simulink model "narx"  (R2019a)
(part 6 of 6)

  "IW{2,1}(60,:)'" : Constant  Value=[0.5846270390584165088654344799579121172428131103515625;0.325648571693005040028623398029594682157039642333984375;-1.1173501219859260924494037681142799556255340576171875;-0.51463684804933806926641182144521735608577728271484375;-0.57361062364307213723435552310547791421413421630859375;-1.3326939837995581683571799658238887786865234375;0.281281193943799745493805630758288316428661346435546875;-0.85669198049516370740974480213481001555919647216796875;0.047948586779547490432928924519728752784430980682373046875;0.90428829582249170560004358776495791971683502197265625]
      mask Display: e = 0.06;c1 = [120 150 230]/255;c2 = ([120 150 230]+0)/383;c3 = ([120 150 230]+128)/383;patch([0 1 1 0],[0 0 1 1],c1);patch([0 1 1 1-e 1-e 0+e],[0 0 1 1-e 0+e 0+e],c2);patch([0 0 1 1-e 0+e 0+e],[0 1 1 1-e 1-e 0+e],c3);plot([0 1 1 0 0],[0 0 1 1 0]);disp('weights');
  "IW{2,1}(61,:)'" : Constant  Value=[0.78103658740860038012243649063748307526111602783203125;1.3860771911427054448040507850237190723419189453125;-0.451371320114015983637756335156154818832874298095703125;-0.335541633513115444831242939471849240362644195556640625;-1.51059236681972119953343280940316617488861083984375;-0.057469963340264003381907542689077672548592090606689453125;1.3584626519773010944192037641187198460102081298828125;-0.629676215555289520153792182100005447864532470703125;-0.60136172032273271792490731968428008258342742919921875;0.9730549079016139746300950719160027801990509033203125]
      mask Display: e = 0.06;c1 = [120 150 230]/255;c2 = ([120 150 230]+0)/383;c3 = ([120 150 230]+128)/383;patch([0 1 1 0],[0 0 1 1],c1);patch([0 1 1 1-e 1-e 0+e],[0 0 1 1-e 0+e 0+e],c2);patch([0 0 1 1-e 0+e 0+e],[0 1 1 1-e 1-e 0+e],c3);plot([0 1 1 0 0],[0 0 1 1 0]);disp('weights');
  "IW{2,1}(62,:)'" : Constant  Value=[0.04940523944418449830973116831955849193036556243896484375;0.63038937153419549730415383237414062023162841796875;-0.400671943461981261425108868934330530464649200439453125;-0.3260626963057704497117583741783164441585540771484375;-1.4699748324566976886984548400505445897579193115234375;-0.52485565032367464954887736894306726753711700439453125;0.52077193033993662840686056370032019913196563720703125;-1.41959117855626715254402370192110538482666015625;-0.61414649132420906507690006037591956555843353271484375;0.9727704163309398577297315569012425839900970458984375]
      mask Display: e = 0.06;c1 = [120 150 230]/255;c2 = ([120 150 230]+0)/383;c3 = ([120 150 230]+128)/383;patch([0 1 1 0],[0 0 1 1],c1);patch([0 1 1 1-e 1-e 0+e],[0 0 1 1-e 0+e 0+e],c2);patch([0 0 1 1-e 0+e 0+e],[0 1 1 1-e 1-e 0+e],c3);plot([0 1 1 0 0],[0 0 1 1 0]);disp('weights');
  "IW{2,1}(63,:)'" : Constant  Value=[0.231719668878419382540556625826866365969181060791015625;0.15579981414367771730411504904623143374919891357421875;-1.133213915627591550361330519081093370914459228515625;-1.01533686843544668221284155151806771755218505859375;-0.5337548818325708044341126878862269222736358642578125;-1.0275630873972179113451375087606720626354217529296875;0.31528407357524856902131205060868524014949798583984375;-0.90450554307037889234521799153299070894718170166015625;-0.80580912230389356576409909393987618386745452880859375;0.902204107924529097317645209841430187225341796875]
      mask Display: e = 0.06;c1 = [120 150 230]/255;c2 = ([120 150 230]+0)/383;c3 = ([120 150 230]+128)/383;patch([0 1 1 0],[0 0 1 1],c1);patch([0 1 1 1-e 1-e 0+e],[0 0 1 1-e 0+e 0+e],c2);patch([0 0 1 1-e 0+e 0+e],[0 1 1 1-e 1-e 0+e],c3);plot([0 1 1 0 0],[0 0 1 1 0]);disp('weights');
  "IW{2,1}(64,:)'" : Constant  Value=[1.0877443347215358659951789377373643219470977783203125;1.193166973587330037531728521571494638919830322265625;-0.42455721543596547373766725286259315907955169677734375;-1.4617036935264919872423661217908374965190887451171875;-1.2080926119362305204418817083933390676975250244140625;-1.0557409686524616976299739690148271620273590087890625;0.365292773089297584387935557970195077359676361083984375;-0.9730446570433100017538663450977765023708343505859375;-0.61090531142060966462992155356914736330509185791015625;0.7703918279306207761436553482781164348125457763671875]
      mask Display: e = 0.06;c1 = [120 150 230]/255;c2 = ([120 150 230]+0)/383;c3 = ([120 150 230]+128)/383;patch([0 1 1 0],[0 0 1 1],c1);patch([0 1 1 1-e 1-e 0+e],[0 0 1 1-e 0+e 0+e],c2);patch([0 0 1 1-e 0+e 0+e],[0 1 1 1-e 1-e 0+e],c3);plot([0 1 1 0 0],[0 0 1 1 0]);disp('weights');
  "IW{2,1}(65,:)'" : Constant  Value=[0.68003601989002981920151569283916614949703216552734375;0.6639319036035191690103829387226141989231109619140625;-0.442406882331512762984715436687110923230648040771484375;-0.55502664647763122474088959279470145702362060546875;-1.43356712752413528733086423017084598541259765625;-0.269969187207295846508969816568423993885517120361328125;1.0574225063279472092148125739186070859432220458984375;-0.78837674667073809331441225367598235607147216796875;-0.5927181169921771353159556383616290986537933349609375;0.93202374184012481972416708231321536004543304443359375]
      mask Display: e = 0.06;c1 = [120 150 230]/255;c2 = ([120 150 230]+0)/383;c3 = ([120 150 230]+128)/383;patch([0 1 1 0],[0 0 1 1],c1);patch([0 1 1 1-e 1-e 0+e],[0 0 1 1-e 0+e 0+e],c2);patch([0 0 1 1-e 0+e 0+e],[0 1 1 1-e 1-e 0+e],c3);plot([0 1 1 0 0],[0 0 1 1 0]);disp('weights');
  "IW{2,1}(66,:)'" : Constant  Value=[0.9744306052910489679419470121501944959163665771484375;0.194329386895280009639463969506323337554931640625;-0.893551305415250407548910516197793185710906982421875;-1.70839989126382629791578438016586005687713623046875;-0.563425857602368740373321998049505054950714111328125;-0.76580929707367972891773888477473519742488861083984375;0.7410351670580634930729502229951322078704833984375;-0.9051439688157305596405421965755522251129150390625;0.024835755139511590805501128897958551533520221710205078125;0.720062910865631788936980228754691779613494873046875]
      mask Display: e = 0.06;c1 = [120 150 230]/255;c2 = ([120 150 230]+0)/383;c3 = ([120 150 230]+128)/383;patch([0 1 1 0],[0 0 1 1],c1);patch([0 1 1 1-e 1-e 0+e],[0 0 1 1-e 0+e 0+e],c2);patch([0 0 1 1-e 0+e 0+e],[0 1 1 1-e 1-e 0+e],c3);plot([0 1 1 0 0],[0 0 1 1 0]);disp('weights');
  "IW{2,1}(67,:)'" : Constant  Value=[0.795900962746471041242557475925423204898834228515625;-1.031300600699818215133518606307916343212127685546875;-0.95195758629597626576668289999361149966716766357421875;-1.2650340176427172789175301659270189702510833740234375;-0.557486607894674079943797551095485687255859375;-0.74762514462963969297248922885046340525150299072265625;0.71583736946448606186521601557615213096141815185546875;-0.89179256466640433043124858158989809453487396240234375;0.221469013754930721393776593686197884380817413330078125;0.77004158983198767174371823784895241260528564453125]
      mask Display: e = 0.06;c1 = [120 150 230]/255;c2 = ([120 150 230]+0)/383;c3 = ([120 150 230]+128)/383;patch([0 1 1 0],[0 0 1 1],c1);patch([0 1 1 1-e 1-e 0+e],[0 0 1 1-e 0+e 0+e],c2);patch([0 0 1 1-e 0+e 0+e],[0 1 1 1-e 1-e 0+e],c3);plot([0 1 1 0 0],[0 0 1 1 0]);disp('weights');
  "IW{2,1}(68,:)'" : Constant  Value=[0.0784208847591110203012476631556637585163116455078125;1.23349585767250236045811107032932341098785400390625;-0.965344275793105222049916847026906907558441162109375;-0.3986454969972170747638529064715839922428131103515625;-0.80448343689417978197297998121939599514007568359375;-0.048251660507535092115016794878101791255176067352294921875;1.217323065165488937822146908729337155818939208984375;-1.253030776061826667699961035395972430706024169921875;0.0162111061744857620769977302188635803759098052978515625;0.96262616564392489149071252541034482419490814208984375]
      mask Display: e = 0.06;c1 = [120 150 230]/255;c2 = ([120 150 230]+0)/383;c3 = ([120 150 230]+128)/383;patch([0 1 1 0],[0 0 1 1],c1);patch([0 1 1 1-e 1-e 0+e],[0 0 1 1-e 0+e 0+e],c2);patch([0 0 1 1-e 0+e 0+e],[0 1 1 1-e 1-e 0+e],c3);plot([0 1 1 0 0],[0 0 1 1 0]);disp('weights');
  "IW{2,1}(69,:)'" : Constant  Value=[0.051272674564019175835749564384968834929168224334716796875;0.43668213391726939942572016661870293319225311279296875;-1.4605052995373946078672133808140642940998077392578125;-1.3530486090437376933692803504527546465396881103515625;-0.189856659347411582672293661744333803653717041015625;-0.91662647122350671136103983371867798268795013427734375;0.7835348999612705700457127022673375904560089111328125;-0.1301188740913402919208152752617024816572666168212890625;-0.80702164776667240086993615477695129811763763427734375;0.91623960712838059539109281104174442589282989501953125]
      mask Display: e = 0.06;c1 = [120 150 230]/255;c2 = ([120 150 230]+0)/383;c3 = ([120 150 230]+128)/383;patch([0 1 1 0],[0 0 1 1],c1);patch([0 1 1 1-e 1-e 0+e],[0 0 1 1-e 0+e 0+e],c2);patch([0 0 1 1-e 0+e 0+e],[0 1 1 1-e 1-e 0+e],c3);plot([0 1 1 0 0],[0 0 1 1 0]);disp('weights');
  "IW{2,1}(7,:)'" : Constant  Value=[-0.074920241317970426297989661179599352180957794189453125;-0.2477101832749133147881792638145270757377147674560546875;-0.78953000952122776023855976745835505425930023193359375;-0.79576047048455311738734963000752031803131103515625;-1.0322962303491272084698948674486018717288970947265625;0.6771202965445819454970433071139268577098846435546875;1.6734147566400012774323613484739325940608978271484375;-0.91740999359185526618176709234830923378467559814453125;-0.89357860194830951439115551693248562514781951904296875;0.9687525516372412770493838252150453627109527587890625]
      mask Display: e = 0.06;c1 = [120 150 230]/255;c2 = ([120 150 230]+0)/383;c3 = ([120 150 230]+128)/383;patch([0 1 1 0],[0 0 1 1],c1);patch([0 1 1 1-e 1-e 0+e],[0 0 1 1-e 0+e 0+e],c2);patch([0 0 1 1-e 0+e 0+e],[0 1 1 1-e 1-e 0+e],c3);plot([0 1 1 0 0],[0 0 1 1 0]);disp('weights');
  "IW{2,1}(70,:)'" : Constant  Value=[0.40830206338846186664426340939826332032680511474609375;1.3423465582091556047572566967573948204517364501953125;-0.594085903064165865572476832312531769275665283203125;-0.98655841293440060812969250036985613405704498291015625;-1.1832782921037701129307606606744229793548583984375;-1.059393468812497740572098336997441947460174560546875;0.3328600660883704875914190779440104961395263671875;-0.85908977292932420244397917485912330448627471923828125;-0.90237675196684852263473430866724811494350433349609375;0.9041786453484832453142416852642782032489776611328125]
      mask Display: e = 0.06;c1 = [120 150 230]/255;c2 = ([120 150 230]+0)/383;c3 = ([120 150 230]+128)/383;patch([0 1 1 0],[0 0 1 1],c1);patch([0 1 1 1-e 1-e 0+e],[0 0 1 1-e 0+e 0+e],c2);patch([0 0 1 1-e 0+e 0+e],[0 1 1 1-e 1-e 0+e],c3);plot([0 1 1 0 0],[0 0 1 1 0]);disp('weights');
  "IW{2,1}(71,:)'" : Constant  Value=[0.683741869146530678591489049722440540790557861328125;1.2893647707153788051215315135777927935123443603515625;-1.25948182914566331191963399760425090789794921875;-1.3331261266872675985695195777225308120250701904296875;-0.376498854306009267389754313626326620578765869140625;-0.8027216540215060813778791271033696830272674560546875;0.72871754596135518422528321025311015546321868896484375;-0.62572871984925415578260299298563040792942047119140625;-0.85659557891590332179276856550131924450397491455078125;0.86199668758921299538400262463255785405635833740234375]
      mask Display: e = 0.06;c1 = [120 150 230]/255;c2 = ([120 150 230]+0)/383;c3 = ([120 150 230]+128)/383;patch([0 1 1 0],[0 0 1 1],c1);patch([0 1 1 1-e 1-e 0+e],[0 0 1 1-e 0+e 0+e],c2);patch([0 0 1 1-e 0+e 0+e],[0 1 1 1-e 1-e 0+e],c3);plot([0 1 1 0 0],[0 0 1 1 0]);disp('weights');
  "IW{2,1}(72,:)'" : Constant  Value=[0.71135244003675091040150846311007626354694366455078125;0.7367893371452252093689594403258524835109710693359375;-0.344668161174500331522807528017438016831874847412109375;-0.480087735884554056564610391433234326541423797607421875;-1.5915567177619303063096367623074911534786224365234375;0.308735582247545325973447916112490929663181304931640625;1.4030786883366257455918457708321511745452880859375;-0.96401773569195781110607867958606220781803131103515625;-0.9150503583203486446251417874009348452091217041015625;0.954110684096918237884210611809976398944854736328125]
      mask Display: e = 0.06;c1 = [120 150 230]/255;c2 = ([120 150 230]+0)/383;c3 = ([120 150 230]+128)/383;patch([0 1 1 0],[0 0 1 1],c1);patch([0 1 1 1-e 1-e 0+e],[0 0 1 1-e 0+e 0+e],c2);patch([0 0 1 1-e 0+e 0+e],[0 1 1 1-e 1-e 0+e],c3);plot([0 1 1 0 0],[0 0 1 1 0]);disp('weights');
  "IW{2,1}(73,:)'" : Constant  Value=[0.4096532059784288026804688342963345348834991455078125;0.41237360182301496802637075234088115394115447998046875;-0.126336401524543617824747343547642230987548828125;-0.414067605535950955530921646641218103468418121337890625;-1.752608967646319459987580557935871183872222900390625;-0.74204868783036292967381086782552301883697509765625;0.5316981000205165397431983365095220506191253662109375;-1.06687302732029110075018252246081829071044921875;-0.342626872137634819193152679872582666575908660888671875;0.929612534888196506699387100525200366973876953125]
      mask Display: e = 0.06;c1 = [120 150 230]/255;c2 = ([120 150 230]+0)/383;c3 = ([120 150 230]+128)/383;patch([0 1 1 0],[0 0 1 1],c1);patch([0 1 1 1-e 1-e 0+e],[0 0 1 1-e 0+e 0+e],c2);patch([0 0 1 1-e 0+e 0+e],[0 1 1 1-e 1-e 0+e],c3);plot([0 1 1 0 0],[0 0 1 1 0]);disp('weights');
  "IW{2,1}(74,:)'" : Constant  Value=[0.66046781455841452324051488176337443292140960693359375;1.195822809542652631620285319513641297817230224609375;-0.01461596518157659563286188131314702332019805908203125;-0.59049806442562891017900028600706718862056732177734375;-1.9183013144081524359307877602986991405487060546875;-0.61136932968790047571161494488478638231754302978515625;0.79859566343875021399156821644282899796962738037109375;-0.71388543526913561532154517408343963325023651123046875;-0.60927724430892293838724071974866092205047607421875;0.92629257542561316274287719352287240326404571533203125]
      mask Display: e = 0.06;c1 = [120 150 230]/255;c2 = ([120 150 230]+0)/383;c3 = ([120 150 230]+128)/383;patch([0 1 1 0],[0 0 1 1],c1);patch([0 1 1 1-e 1-e 0+e],[0 0 1 1-e 0+e 0+e],c2);patch([0 0 1 1-e 0+e 0+e],[0 1 1 1-e 1-e 0+e],c3);plot([0 1 1 0 0],[0 0 1 1 0]);disp('weights');
  "IW{2,1}(75,:)'" : Constant  Value=[0.2438183207692106446717872358931344933807849884033203125;1.032272957592475837174106345628388226032257080078125;-0.7374303641036608070180591312237083911895751953125;-0.80593752511152672024508092363248579204082489013671875;-1.0045024970739448999523801830946467816829681396484375;-1.393856540491007489634966987068764865398406982421875;0.08664968480477412693385730335648986510932445526123046875;-0.91717442950897953846123300536419264972209930419921875;-0.52637328782331171961317295426852069795131683349609375;0.91253498567823199127957423115731216967105865478515625]
      mask Display: e = 0.06;c1 = [120 150 230]/255;c2 = ([120 150 230]+0)/383;c3 = ([120 150 230]+128)/383;patch([0 1 1 0],[0 0 1 1],c1);patch([0 1 1 1-e 1-e 0+e],[0 0 1 1-e 0+e 0+e],c2);patch([0 0 1 1-e 0+e 0+e],[0 1 1 1-e 1-e 0+e],c3);plot([0 1 1 0 0],[0 0 1 1 0]);disp('weights');
  "IW{2,1}(76,:)'" : Constant  Value=[0.09687738069406558183427335961823700927197933197021484375;0.0671463051349393269529031158526777289807796478271484375;-0.75187637360477210801690262087504379451274871826171875;-0.2286881485536169378303128496554563753306865692138671875;-1.1094798811126265203341745291254483163356781005859375;-0.5083855113551345450417784377350471913814544677734375;0.76877004074804322630853903319803066551685333251953125;-0.97804707781086175355511613815906457602977752685546875;-0.380452406263650899642669855893473140895366668701171875;0.991968038311260347228426326182670891284942626953125]
      mask Display: e = 0.06;c1 = [120 150 230]/255;c2 = ([120 150 230]+0)/383;c3 = ([120 150 230]+128)/383;patch([0 1 1 0],[0 0 1 1],c1);patch([0 1 1 1-e 1-e 0+e],[0 0 1 1-e 0+e 0+e],c2);patch([0 0 1 1-e 0+e 0+e],[0 1 1 1-e 1-e 0+e],c3);plot([0 1 1 0 0],[0 0 1 1 0]);disp('weights');
  "IW{2,1}(77,:)'" : Constant  Value=[0.698276902011685240978522415389306843280792236328125;-1.201074382401174034384894184768199920654296875;-0.1909041138723935049359425875081797130405902862548828125;-0.98721006380672149393973313635797239840030670166015625;-1.443656037243777223721963309799320995807647705078125;0.0238991493223953098412604134637149400077760219573974609375;0.98515016863503468425022902010823599994182586669921875;-1.53867215379339317138374099158681929111480712890625;0.0904827129009844188800570918829180300235748291015625;0.7856307163361719858585274778306484222412109375]
      mask Display: e = 0.06;c1 = [120 150 230]/255;c2 = ([120 150 230]+0)/383;c3 = ([120 150 230]+128)/383;patch([0 1 1 0],[0 0 1 1],c1);patch([0 1 1 1-e 1-e 0+e],[0 0 1 1-e 0+e 0+e],c2);patch([0 0 1 1-e 0+e 0+e],[0 1 1 1-e 1-e 0+e],c3);plot([0 1 1 0 0],[0 0 1 1 0]);disp('weights');
  "IW{2,1}(78,:)'" : Constant  Value=[0.62253311758509310980258533163578249514102935791015625;-0.98911649688906688737688455148600041866302490234375;-0.94230752757691249588134496661950834095478057861328125;-0.59448134893245185850219058920629322528839111328125;-0.69601449228161726967556433010031469166278839111328125;-1.53769269557400178882744512520730495452880859375;0.1449914530402906798212114836132968775928020477294921875;-0.72814111352036980928659204437281005084514617919921875;0.4110419113490182407844031331478618085384368896484375;0.85859744277036675885739214209024794399738311767578125]
      mask Display: e = 0.06;c1 = [120 150 230]/255;c2 = ([120 150 230]+0)/383;c3 = ([120 150 230]+128)/383;patch([0 1 1 0],[0 0 1 1],c1);patch([0 1 1 1-e 1-e 0+e],[0 0 1 1-e 0+e 0+e],c2);patch([0 0 1 1-e 0+e 0+e],[0 1 1 1-e 1-e 0+e],c3);plot([0 1 1 0 0],[0 0 1 1 0]);disp('weights');
  "IW{2,1}(79,:)'" : Constant  Value=[0.043504837709850092963836942772104521282017230987548828125;-0.881793197855445409771846243529580533504486083984375;-0.70598483564032654680175937755848281085491180419921875;0.0347001328854996959893952634956804104149341583251953125;-1.1911737829599682303438612507306970655918121337890625;-0.42973335414514857166778938335482962429523468017578125;0.75247005926979848577929033126565627753734588623046875;-1.036034229685881324911633782903663814067840576171875;-0.32316180089984014589532534955651499330997467041015625;1.014762120153226643282096119946800172328948974609375]
      mask Display: e = 0.06;c1 = [120 150 230]/255;c2 = ([120 150 230]+0)/383;c3 = ([120 150 230]+128)/383;patch([0 1 1 0],[0 0 1 1],c1);patch([0 1 1 1-e 1-e 0+e],[0 0 1 1-e 0+e 0+e],c2);patch([0 0 1 1-e 0+e 0+e],[0 1 1 1-e 1-e 0+e],c3);plot([0 1 1 0 0],[0 0 1 1 0]);disp('weights');
  "IW{2,1}(8,:)'" : Constant  Value=[0.59887455435518088808777292797458358108997344970703125;1.0842680808772076073154266850906424224376678466796875;-1.1599765734110014658853060609544627368450164794921875;-0.701460341813013865674975022557191550731658935546875;-0.66671728212999215035239330973126925528049468994140625;-0.4305914240781938406854578715865500271320343017578125;1.1580928678115733898579264860018156468868255615234375;-0.333742483642422260725624028054880909621715545654296875;-0.67987921675175611024855015784851275384426116943359375;0.96448277176620200723533571363077498972415924072265625]
      mask Display: e = 0.06;c1 = [120 150 230]/255;c2 = ([120 150 230]+0)/383;c3 = ([120 150 230]+128)/383;patch([0 1 1 0],[0 0 1 1],c1);patch([0 1 1 1-e 1-e 0+e],[0 0 1 1-e 0+e 0+e],c2);patch([0 0 1 1-e 0+e 0+e],[0 1 1 1-e 1-e 0+e],c3);plot([0 1 1 0 0],[0 0 1 1 0]);disp('weights');
  "IW{2,1}(80,:)'" : Constant  Value=[0.15125446175658863179336321991286240518093109130859375;0.57772564222751199292105184213141910731792449951171875;-0.86182323778516767287527500229771248996257781982421875;-1.0635023193803767593834663784946314990520477294921875;-0.735646891627312893291446016519330441951751708984375;-1.2761082798077694189231579002807848155498504638671875;0.2450391375786898640054545239763683639466762542724609375;-1.0213315809567411474034770435537211596965789794921875;0.084759263924596706107905674798530526459217071533203125;0.8505132244778821348774044963647611439228057861328125]
      mask Display: e = 0.06;c1 = [120 150 230]/255;c2 = ([120 150 230]+0)/383;c3 = ([120 150 230]+128)/383;patch([0 1 1 0],[0 0 1 1],c1);patch([0 1 1 1-e 1-e 0+e],[0 0 1 1-e 0+e 0+e],c2);patch([0 0 1 1-e 0+e 0+e],[0 1 1 1-e 1-e 0+e],c3);plot([0 1 1 0 0],[0 0 1 1 0]);disp('weights');
  "IW{2,1}(81,:)'" : Constant  Value=[1.1069833850167258848529172610142268240451812744140625;1.870671312385265849798088311217725276947021484375;-0.33099715440554378087512077399878762662410736083984375;-0.8340741057726452911680325996712781488895416259765625;-1.4939414108250428370183726656250655651092529296875;-1.0227305771095605013698559559998102486133575439453125;0.48391307819007256529886262796935625374317169189453125;-0.808134471975317847380892999353818595409393310546875;-0.6794702636326206413031059128115884959697723388671875;0.87009885498775652035163830078090541064739227294921875]
      mask Display: e = 0.06;c1 = [120 150 230]/255;c2 = ([120 150 230]+0)/383;c3 = ([120 150 230]+128)/383;patch([0 1 1 0],[0 0 1 1],c1);patch([0 1 1 1-e 1-e 0+e],[0 0 1 1-e 0+e 0+e],c2);patch([0 0 1 1-e 0+e 0+e],[0 1 1 1-e 1-e 0+e],c3);plot([0 1 1 0 0],[0 0 1 1 0]);disp('weights');
  "IW{2,1}(82,:)'" : Constant  Value=[0.215034771223415244190135808821651153266429901123046875;-0.371362786379315468199280303451814688742160797119140625;-0.649145927683384638129382437909953296184539794921875;-0.8107093968121394933490364564931951463222503662109375;-1.1108466174022886274741495071793906390666961669921875;-0.448898693785944880030314152463688515126705169677734375;0.77418260161640362060353481865604408085346221923828125;-0.9218841214205715228757753720856271684169769287109375;-0.5764798905729924261009955444023944437503814697265625;0.91286956848360734095848556535202078521251678466796875]
      mask Display: e = 0.06;c1 = [120 150 230]/255;c2 = ([120 150 230]+0)/383;c3 = ([120 150 230]+128)/383;patch([0 1 1 0],[0 0 1 1],c1);patch([0 1 1 1-e 1-e 0+e],[0 0 1 1-e 0+e 0+e],c2);patch([0 0 1 1-e 0+e 0+e],[0 1 1 1-e 1-e 0+e],c3);plot([0 1 1 0 0],[0 0 1 1 0]);disp('weights');
  "IW{2,1}(83,:)'" : Constant  Value=[0.735006465514477014266958576627075672149658203125;0.7732649327048755072411267974530346691608428955078125;-0.267233584913366239987908556940965354442596435546875;0.0111084397578394798722367653454057290218770503997802734375;-1.59738900655409832296527383732609450817108154296875;-1.002082661993780821063637631596066057682037353515625;0.18815659312723698182168163839378394186496734619140625;-1.5841358909757599082723800165695138275623321533203125;-0.08745941188448962122503616001267801038920879364013671875;0.93039645817548788375717094822903163731098175048828125]
      mask Display: e = 0.06;c1 = [120 150 230]/255;c2 = ([120 150 230]+0)/383;c3 = ([120 150 230]+128)/383;patch([0 1 1 0],[0 0 1 1],c1);patch([0 1 1 1-e 1-e 0+e],[0 0 1 1-e 0+e 0+e],c2);patch([0 0 1 1-e 0+e 0+e],[0 1 1 1-e 1-e 0+e],c3);plot([0 1 1 0 0],[0 0 1 1 0]);disp('weights');
  "IW{2,1}(84,:)'" : Constant  Value=[0.66569584992328512118575645217788405716419219970703125;-0.092187130897322611122746138789807446300983428955078125;-0.348810099764139625033720903957146219909191131591796875;-1.14363673480168781537713584839366376399993896484375;-1.3349635928639020931996128638274967670440673828125;-0.892557166096453524772869059233926236629486083984375;0.404140910762284588653159289606264792382717132568359375;-1.0096866012918030985900941232102923095226287841796875;-0.462454601830129152784110146967577748000621795654296875;0.8197709706988567379681853708461858332157135009765625]
      mask Display: e = 0.06;c1 = [120 150 230]/255;c2 = ([120 150 230]+0)/383;c3 = ([120 150 230]+128)/383;patch([0 1 1 0],[0 0 1 1],c1);patch([0 1 1 1-e 1-e 0+e],[0 0 1 1-e 0+e 0+e],c2);patch([0 0 1 1-e 0+e 0+e],[0 1 1 1-e 1-e 0+e],c3);plot([0 1 1 0 0],[0 0 1 1 0]);disp('weights');
  "IW{2,1}(85,:)'" : Constant  Value=[0.8712401316466877876365515476209111511707305908203125;-0.76879853949288434744602227510767988860607147216796875;-1.265795754406632500632667870377190411090850830078125;-0.73570648832773921643735093311988748610019683837890625;-0.338488477364097650745833334440249018371105194091796875;-1.055919737994191809349331379053182899951934814453125;0.479437482323288699515018151942058466374874114990234375;-0.83568296206173353635193734589847736060619354248046875;0.031986522995903689248198276118273497559130191802978515625;0.85081109880058647387812698070774786174297332763671875]
      mask Display: e = 0.06;c1 = [120 150 230]/255;c2 = ([120 150 230]+0)/383;c3 = ([120 150 230]+128)/383;patch([0 1 1 0],[0 0 1 1],c1);patch([0 1 1 1-e 1-e 0+e],[0 0 1 1-e 0+e 0+e],c2);patch([0 0 1 1-e 0+e 0+e],[0 1 1 1-e 1-e 0+e],c3);plot([0 1 1 0 0],[0 0 1 1 0]);disp('weights');
  "IW{2,1}(86,:)'" : Constant  Value=[0.78825913226714805492889581728377379477024078369140625;0.79549621499637301891283414079225622117519378662109375;-0.80100420096192259666878499047015793621540069580078125;-1.052614336778985748566128677339293062686920166015625;-1.0048393985698116370741672653821296989917755126953125;-1.40601029551436429443356246338225901126861572265625;0.362987678205423491828440774042974226176738739013671875;-0.04781798311889333408242208633964764885604381561279296875;-1.049253314017066340824158032773993909358978271484375;0.90589665862637158699754991175723262131214141845703125]
      mask Display: e = 0.06;c1 = [120 150 230]/255;c2 = ([120 150 230]+0)/383;c3 = ([120 150 230]+128)/383;patch([0 1 1 0],[0 0 1 1],c1);patch([0 1 1 1-e 1-e 0+e],[0 0 1 1-e 0+e 0+e],c2);patch([0 0 1 1-e 0+e 0+e],[0 1 1 1-e 1-e 0+e],c3);plot([0 1 1 0 0],[0 0 1 1 0]);disp('weights');
  "IW{2,1}(87,:)'" : Constant  Value=[0.32216607457254042845562480579246766865253448486328125;0.93104270543261247183863815735094249248504638671875;-0.6249835442353168790674544652574695646762847900390625;-0.926713305141846799273253054707311093807220458984375;-1.2339118409345692928269500043825246393680572509765625;0.2308094410376762828374097580308443866670131683349609375;1.4019202901908627278970698171178810298442840576171875;-0.74068417963864607855839494732208549976348876953125;-1.1384985749521099318570804825867526233196258544921875;0.94888315687380153651275804804754443466663360595703125]
      mask Display: e = 0.06;c1 = [120 150 230]/255;c2 = ([120 150 230]+0)/383;c3 = ([120 150 230]+128)/383;patch([0 1 1 0],[0 0 1 1],c1);patch([0 1 1 1-e 1-e 0+e],[0 0 1 1-e 0+e 0+e],c2);patch([0 0 1 1-e 0+e 0+e],[0 1 1 1-e 1-e 0+e],c3);plot([0 1 1 0 0],[0 0 1 1 0]);disp('weights');
  "IW{2,1}(88,:)'" : Constant  Value=[0.2319380511292025437430908141323016025125980377197265625;-0.3809134658308404031146210400038398802280426025390625;-1.6437841061874689518873537963372655212879180908203125;-0.9725254218160805930182277734274975955486297607421875;-0.056490275535695626263343882556000608019530773162841796875;-0.51773751634603104587739608177798800170421600341796875;1.1344178065922527753883741752360947430133819580078125;-0.07293239459924523437894805510950391180813312530517578125;-0.71606183580065174698603414071840234100818634033203125;0.95233094118410954731501760761602781713008880615234375]
      mask Display: e = 0.06;c1 = [120 150 230]/255;c2 = ([120 150 230]+0)/383;c3 = ([120 150 230]+128)/383;patch([0 1 1 0],[0 0 1 1],c1);patch([0 1 1 1-e 1-e 0+e],[0 0 1 1-e 0+e 0+e],c2);patch([0 0 1 1-e 0+e 0+e],[0 1 1 1-e 1-e 0+e],c3);plot([0 1 1 0 0],[0 0 1 1 0]);disp('weights');
  "IW{2,1}(89,:)'" : Constant  Value=[0.792533746222353396859716667677275836467742919921875;-0.1219775428896825442137696882127784192562103271484375;-0.6904996306424704410886761252186261117458343505859375;-0.941758692375770589677586031029932200908660888671875;-0.905836517768802362837732289335690438747406005859375;-1.4526052872247114944315171669586561620235443115234375;0.000584171061013600612966956138194518644013442099094390869140625;-1.162966647957240251542998521472327411174774169921875;0.061679374632315743520738493543831282295286655426025390625;0.80408855442849735961630130987032316625118255615234375]
      mask Display: e = 0.06;c1 = [120 150 230]/255;c2 = ([120 150 230]+0)/383;c3 = ([120 150 230]+128)/383;patch([0 1 1 0],[0 0 1 1],c1);patch([0 1 1 1-e 1-e 0+e],[0 0 1 1-e 0+e 0+e],c2);patch([0 0 1 1-e 0+e 0+e],[0 1 1 1-e 1-e 0+e],c3);plot([0 1 1 0 0],[0 0 1 1 0]);disp('weights');
  "IW{2,1}(9,:)'" : Constant  Value=[1.3354366427815460571792982591432519257068634033203125;-0.629343904052440894503206436638720333576202392578125;-0.9060459906264519691632131070946343243122100830078125;-1.855680002744634737865681017865426838397979736328125;-0.323768235929574432763189406614401377737522125244140625;-0.83572193646278503109670054982416331768035888671875;0.6980391343872967002681662052054889500141143798828125;-1.349731997878071521057563586509786546230316162109375;0.74653958435369471846598798947525210678577423095703125;0.58583964960055745496703138996963389217853546142578125]
      mask Display: e = 0.06;c1 = [120 150 230]/255;c2 = ([120 150 230]+0)/383;c3 = ([120 150 230]+128)/383;patch([0 1 1 0],[0 0 1 1],c1);patch([0 1 1 1-e 1-e 0+e],[0 0 1 1-e 0+e 0+e],c2);patch([0 0 1 1-e 0+e 0+e],[0 1 1 1-e 1-e 0+e],c3);plot([0 1 1 0 0],[0 0 1 1 0]);disp('weights');
  "IW{2,1}(90,:)'" : Constant  Value=[0.59092120144319093544282850416493602097034454345703125;0.38549453104067221698159073639544658362865447998046875;-1.5320913413474956943360894001671113073825836181640625;-1.244862148363711895626693149097263813018798828125;-0.050598275569687045649658330148668028414249420166015625;-0.89188177096418286282641929574310779571533203125;0.59258716478466022525850576130324043333530426025390625;-0.70729304174109219882637944465386681258678436279296875;-0.7600987662816738321680531953461468219757080078125;0.86542221733170021646941449944279156625270843505859375]
      mask Display: e = 0.06;c1 = [120 150 230]/255;c2 = ([120 150 230]+0)/383;c3 = ([120 150 230]+128)/383;patch([0 1 1 0],[0 0 1 1],c1);patch([0 1 1 1-e 1-e 0+e],[0 0 1 1-e 0+e 0+e],c2);patch([0 0 1 1-e 0+e 0+e],[0 1 1 1-e 1-e 0+e],c3);plot([0 1 1 0 0],[0 0 1 1 0]);disp('weights');
  "IW{2,1}(91,:)'" : Constant  Value=[0.069311670468534425371132101645343936979770660400390625;-0.166519237161024180604584898901521228253841400146484375;-1.0208774047940443185922276825294829905033111572265625;-0.3660977655542347886097331866039894521236419677734375;-0.57286734817648454765048882109113037586212158203125;-0.892778913174406607566879756632260978221893310546875;0.243887459662816385996819690262782387435436248779296875;-1.8821316397728080627160807125619612634181976318359375;0.53306510054586364599771286520990543067455291748046875;0.887817741656797831950598265393637120723724365234375]
      mask Display: e = 0.06;c1 = [120 150 230]/255;c2 = ([120 150 230]+0)/383;c3 = ([120 150 230]+128)/383;patch([0 1 1 0],[0 0 1 1],c1);patch([0 1 1 1-e 1-e 0+e],[0 0 1 1-e 0+e 0+e],c2);patch([0 0 1 1-e 0+e 0+e],[0 1 1 1-e 1-e 0+e],c3);plot([0 1 1 0 0],[0 0 1 1 0]);disp('weights');
  "IW{2,1}(92,:)'" : Constant  Value=[0.0184006715237334909918143210916241514496505260467529296875;-0.2701310809544790192404661866021342575550079345703125;-1.0921154944258144592339476730558089911937713623046875;-1.224546257081914557574009450036101043224334716796875;-0.6230406348119672532703816614230163395404815673828125;-1.1981601655552684970729160340852104127407073974609375;0.4724395220614219237376119053806178271770477294921875;-0.07933870033885280503849202204946777783334255218505859375;-0.8896646976242965632053483204799704253673553466796875;0.9231905129560205036653997012763284146785736083984375]
      mask Display: e = 0.06;c1 = [120 150 230]/255;c2 = ([120 150 230]+0)/383;c3 = ([120 150 230]+128)/383;patch([0 1 1 0],[0 0 1 1],c1);patch([0 1 1 1-e 1-e 0+e],[0 0 1 1-e 0+e 0+e],c2);patch([0 0 1 1-e 0+e 0+e],[0 1 1 1-e 1-e 0+e],c3);plot([0 1 1 0 0],[0 0 1 1 0]);disp('weights');
  "IW{2,1}(93,:)'" : Constant  Value=[0.62270166073915589333154230189393274486064910888671875;0.1977310314279116243429967880729236640036106109619140625;-0.9526316945427797389100987857091240584850311279296875;-1.1212923287608587141761518068960867822170257568359375;-0.69835181966180714940861662398674525320529937744140625;-0.41840016053703521503592810404370538890361785888671875;0.98029982377078661581748519893153570592403411865234375;-0.79557109896550637362366842353367246687412261962890625;-0.3815569023232920908839105322840623557567596435546875;0.85249484437307232465030892853974364697933197021484375]
      mask Display: e = 0.06;c1 = [120 150 230]/255;c2 = ([120 150 230]+0)/383;c3 = ([120 150 230]+128)/383;patch([0 1 1 0],[0 0 1 1],c1);patch([0 1 1 1-e 1-e 0+e],[0 0 1 1-e 0+e 0+e],c2);patch([0 0 1 1-e 0+e 0+e],[0 1 1 1-e 1-e 0+e],c3);plot([0 1 1 0 0],[0 0 1 1 0]);disp('weights');
  "IW{2,1}(94,:)'" : Constant  Value=[0.321117519912699822537405225375550799071788787841796875;-0.732732290619085180338743157335557043552398681640625;-0.84028374883293455166466401351499371230602264404296875;-1.71465841745636993209700449369847774505615234375;-0.7696069549049810998297971309511922299861907958984375;-0.73060386298644741653873779796413145959377288818359375;0.7299139882172849258523683602106757462024688720703125;-0.327146330225191406260165649655391462147235870361328125;-0.888474413431640019922497231164015829563140869140625;0.82318630265610248653018743425491265952587127685546875]
      mask Display: e = 0.06;c1 = [120 150 230]/255;c2 = ([120 150 230]+0)/383;c3 = ([120 150 230]+128)/383;patch([0 1 1 0],[0 0 1 1],c1);patch([0 1 1 1-e 1-e 0+e],[0 0 1 1-e 0+e 0+e],c2);patch([0 0 1 1-e 0+e 0+e],[0 1 1 1-e 1-e 0+e],c3);plot([0 1 1 0 0],[0 0 1 1 0]);disp('weights');
  "IW{2,1}(95,:)'" : Constant  Value=[-0.18330285839000037828583344889921136200428009033203125;1.417763617976048440283420859486795961856842041015625;-0.7506975077638440296823318931274116039276123046875;-0.20843487546265981880111439750180579721927642822265625;-1.2343130017710495227589717615046538412570953369140625;-0.289557015219637226000060081787523813545703887939453125;0.94238166364007935893454259712598286569118499755859375;-0.8562725145497005474481966302846558392047882080078125;-1.03967969220242206773718862677924335002899169921875;1.0687727006662097739564387666177935898303985595703125]
      mask Display: e = 0.06;c1 = [120 150 230]/255;c2 = ([120 150 230]+0)/383;c3 = ([120 150 230]+128)/383;patch([0 1 1 0],[0 0 1 1],c1);patch([0 1 1 1-e 1-e 0+e],[0 0 1 1-e 0+e 0+e],c2);patch([0 0 1 1-e 0+e 0+e],[0 1 1 1-e 1-e 0+e],c3);plot([0 1 1 0 0],[0 0 1 1 0]);disp('weights');
  "IW{2,1}(96,:)'" : Constant  Value=[0.69644878128478138190615709390840493142604827880859375;0.123270978372166606362725360668264329433441162109375;0.1749176767156547518400344642941490747034549713134765625;-0.315389058266458022217193502001464366912841796875;-2.128807425271676212474858402856625616550445556640625;-1.329976205804500377638532881974242627620697021484375;0.01505491976050171536172239683537554810754954814910888671875;-0.89365983606735011068877838624757714569568634033203125;-0.65492254508844982563431358357775025069713592529296875;0.9284164937412155982343620053143240511417388916015625]
      mask Display: e = 0.06;c1 = [120 150 230]/255;c2 = ([120 150 230]+0)/383;c3 = ([120 150 230]+128)/383;patch([0 1 1 0],[0 0 1 1],c1);patch([0 1 1 1-e 1-e 0+e],[0 0 1 1-e 0+e 0+e],c2);patch([0 0 1 1-e 0+e 0+e],[0 1 1 1-e 1-e 0+e],c3);plot([0 1 1 0 0],[0 0 1 1 0]);disp('weights');
  "IW{2,1}(97,:)'" : Constant  Value=[-0.1045902401669992765054217898068600334227085113525390625;0.69147561526502088202761342472513206303119659423828125;-0.454550610681903888288246662341407500207424163818359375;-0.69830923014718748742524212502758018672466278076171875;-1.4812378684536320339049098038231022655963897705078125;0.407749506455176824459840645431540906429290771484375;1.5131776815029265303991223845514468848705291748046875;-0.744788679380567142374047762132249772548675537109375;-1.0766619728685480339436253416351974010467529296875;1.0017313917205641349283951058168895542621612548828125]
      mask Display: e = 0.06;c1 = [120 150 230]/255;c2 = ([120 150 230]+0)/383;c3 = ([120 150 230]+128)/383;patch([0 1 1 0],[0 0 1 1],c1);patch([0 1 1 1-e 1-e 0+e],[0 0 1 1-e 0+e 0+e],c2);patch([0 0 1 1-e 0+e 0+e],[0 1 1 1-e 1-e 0+e],c3);plot([0 1 1 0 0],[0 0 1 1 0]);disp('weights');
  "IW{2,1}(98,:)'" : Constant  Value=[0.09843633709816158872119018496960052289068698883056640625;-1.00348089629137415812465405906550586223602294921875;-0.09980628032932560567136448526071035303175449371337890625;-1.1801195107314461640868330505327321588993072509765625;-1.6213484900120753717800425874884240329265594482421875;-0.62213767320548207795383177654002793133258819580078125;0.6000939534283189491503662793547846376895904541015625;-0.86922162235170408184359303049859590828418731689453125;-0.39607703919225178967877809554920531809329986572265625;0.84684781018750110437309785993420518934726715087890625]
      mask Display: e = 0.06;c1 = [120 150 230]/255;c2 = ([120 150 230]+0)/383;c3 = ([120 150 230]+128)/383;patch([0 1 1 0],[0 0 1 1],c1);patch([0 1 1 1-e 1-e 0+e],[0 0 1 1-e 0+e 0+e],c2);patch([0 0 1 1-e 0+e 0+e],[0 1 1 1-e 1-e 0+e],c3);plot([0 1 1 0 0],[0 0 1 1 0]);disp('weights');
  "IW{2,1}(99,:)'" : Constant  Value=[0.2255310748738143800107280867450754158198833465576171875;0.0582861152635134605048961020656861364841461181640625;-1.1815578728791320539670550715527497231960296630859375;-0.747580828657393059444302707561291754245758056640625;-0.52811898564728132487999801014666445553302764892578125;0.37177678522365120716841602188651449978351593017578125;1.3429840855392971565862580973771400749683380126953125;-1.31747915115486335935202077962458133697509765625;-0.70203951001937403564312489834264852106571197509765625;0.93351517917566884108282465604133903980255126953125]
      mask Display: e = 0.06;c1 = [120 150 230]/255;c2 = ([120 150 230]+0)/383;c3 = ([120 150 230]+128)/383;patch([0 1 1 0],[0 0 1 1],c1);patch([0 1 1 1-e 1-e 0+e],[0 0 1 1-e 0+e 0+e],c2);patch([0 0 1 1-e 0+e 0+e],[0 1 1 1-e 1-e 0+e],c3);plot([0 1 1 0 0],[0 0 1 1 0]);disp('weights');
  Mux : Mux  Inputs=200
      mask Display: e = 0.06;c1 = [120 150 230]/255;c2 = ([120 150 230]+0)/383;c3 = ([120 150 230]+128)/383;patch([0 1 1 0],[0 0 1 1],c1);patch([0 1 1 1-e 1-e 0+e],[0 0 1 1-e 0+e 0+e],c2);patch([0 0 1 1-e 0+e 0+e],[0 1 1 1-e 1-e 0+e],c3);plot([0 1 1 0 0],[0 0 1 1 0]);disp('Mux');
  dotprod{1..200} (200 alike) : neural/Weight Functions/dotprod
      settings: SourceProductName=MATLAB Runtime - Deep Learning Toolbox  SourceProductBaseCode=Missing
  "lz{2,1}" : Outport
      mask Display: e = 0.06;c1 = [120 230 180]/255;c2 = ([120 230 180]+0)/(256+128);c3 = ([120 230 180]+128)/(256+128);patch([0 1 1 0],[0 0 1 1],c1);patch([0 1 1 1-e 1-e 0+e],[0 0 1 1-e 0+e 0+e],c2);patch([0 0 1 1-e 0+e 0+e],[0 1 1 1-e 1-e 0+e],c3);plot([0 1 1 0 0],[0 0 1 1 0]);
  wires:
  "IW{2,1}(1,:)'"/1 -> dotprod1/1
  "ad{2,1}"/1 -> dotprod1/2, dotprod2/2, dotprod3/2, dotprod4/2, dotprod5/2, dotprod6/2, dotprod7/2, dotprod8/2, dotprod9/2, dotprod10/2, dotprod11/2, dotprod12/2, dotprod13/2, dotprod14/2, dotprod15/2, dotprod16/2, dotprod17/2, dotprod18/2, dotprod19/2, dotprod20/2, dotprod21/2, dotprod22/2, dotprod23/2, dotprod24/2, dotprod25/2, dotprod26/2, dotprod27/2, dotprod28/2, dotprod29/2, dotprod30/2, dotprod31/2, dotprod32/2, dotprod33/2, dotprod34/2, dotprod35/2, dotprod36/2, dotprod37/2, dotprod38/2, dotprod39/2, dotprod40/2, dotprod41/2, dotprod42/2, dotprod43/2, dotprod44/2, dotprod45/2, dotprod46/2, dotprod47/2, dotprod48/2, dotprod49/2, dotprod50/2, dotprod51/2, dotprod52/2, dotprod53/2, dotprod54/2, dotprod55/2, dotprod56/2, dotprod57/2, dotprod58/2, dotprod59/2, dotprod60/2, dotprod61/2, dotprod62/2, dotprod63/2, dotprod64/2, dotprod65/2, dotprod66/2, dotprod67/2, dotprod68/2, dotprod69/2, dotprod70/2, dotprod71/2, dotprod72/2, dotprod73/2, dotprod74/2, dotprod75/2, dotprod76/2, dotprod77/2, dotprod78/2, dotprod79/2, dotprod80/2, dotprod81/2, dotprod82/2, dotprod83/2, dotprod84/2, dotprod85/2, dotprod86/2, dotprod87/2, dotprod88/2, dotprod89/2, dotprod90/2, dotprod91/2, dotprod92/2, dotprod93/2, dotprod94/2, dotprod95/2, dotprod96/2, dotprod97/2, dotprod98/2, dotprod99/2, dotprod100/2, dotprod101/2, dotprod102/2, dotprod103/2, dotprod104/2, dotprod105/2, dotprod106/2, dotprod107/2, dotprod108/2, dotprod109/2, dotprod110/2, dotprod111/2, dotprod112/2, dotprod113/2, dotprod114/2, dotprod115/2, dotprod116/2, dotprod117/2, dotprod118/2, dotprod119/2, dotprod120/2, dotprod121/2, dotprod122/2, dotprod123/2, dotprod124/2, dotprod125/2, dotprod126/2, dotprod127/2, dotprod128/2, dotprod129/2, dotprod130/2, dotprod131/2, dotprod132/2, dotprod133/2, dotprod134/2, dotprod135/2, dotprod136/2, dotprod137/2, dotprod138/2, dotprod139/2, dotprod140/2, dotprod141/2, dotprod142/2, dotprod143/2, dotprod144/2, dotprod145/2, dotprod146/2, dotprod147/2, dotprod148/2, dotprod149/2, dotprod150/2, dotprod151/2, dotprod152/2, dotprod153/2, dotprod154/2, dotprod155/2, dotprod156/2, dotprod157/2, dotprod158/2, dotprod159/2, dotprod160/2, dotprod161/2, dotprod162/2, dotprod163/2, dotprod164/2, dotprod165/2, dotprod166/2, dotprod167/2, dotprod168/2, dotprod169/2, dotprod170/2, dotprod171/2, dotprod172/2, dotprod173/2, dotprod174/2, dotprod175/2, dotprod176/2, dotprod177/2, dotprod178/2, dotprod179/2, dotprod180/2, dotprod181/2, dotprod182/2, dotprod183/2, dotprod184/2, dotprod185/2, dotprod186/2, dotprod187/2, dotprod188/2, dotprod189/2, dotprod190/2, dotprod191/2, dotprod192/2, dotprod193/2, dotprod194/2, dotprod195/2, dotprod196/2, dotprod197/2, dotprod198/2, dotprod199/2, dotprod200/2
  dotprod1/1 -> Mux/1
  "IW{2,1}(2,:)'"/1 -> dotprod2/1
  dotprod2/1 -> Mux/2
  "IW{2,1}(3,:)'"/1 -> dotprod3/1
  dotprod3/1 -> Mux/3
  "IW{2,1}(4,:)'"/1 -> dotprod4/1
  dotprod4/1 -> Mux/4
  "IW{2,1}(5,:)'"/1 -> dotprod5/1
  dotprod5/1 -> Mux/5
  "IW{2,1}(6,:)'"/1 -> dotprod6/1
  dotprod6/1 -> Mux/6
  "IW{2,1}(7,:)'"/1 -> dotprod7/1
  dotprod7/1 -> Mux/7
  "IW{2,1}(8,:)'"/1 -> dotprod8/1
  dotprod8/1 -> Mux/8
  "IW{2,1}(9,:)'"/1 -> dotprod9/1
  dotprod9/1 -> Mux/9
  "IW{2,1}(10,:)'"/1 -> dotprod10/1
  dotprod10/1 -> Mux/10
  "IW{2,1}(11,:)'"/1 -> dotprod11/1
  dotprod11/1 -> Mux/11
  "IW{2,1}(12,:)'"/1 -> dotprod12/1
  dotprod12/1 -> Mux/12
  "IW{2,1}(13,:)'"/1 -> dotprod13/1
  dotprod13/1 -> Mux/13
  "IW{2,1}(14,:)'"/1 -> dotprod14/1
  dotprod14/1 -> Mux/14
  "IW{2,1}(15,:)'"/1 -> dotprod15/1
  dotprod15/1 -> Mux/15
  "IW{2,1}(16,:)'"/1 -> dotprod16/1
  dotprod16/1 -> Mux/16
  "IW{2,1}(17,:)'"/1 -> dotprod17/1
  dotprod17/1 -> Mux/17
  "IW{2,1}(18,:)'"/1 -> dotprod18/1
  dotprod18/1 -> Mux/18
  "IW{2,1}(19,:)'"/1 -> dotprod19/1
  dotprod19/1 -> Mux/19
  "IW{2,1}(20,:)'"/1 -> dotprod20/1
  dotprod20/1 -> Mux/20
  "IW{2,1}(21,:)'"/1 -> dotprod21/1
  dotprod21/1 -> Mux/21
  "IW{2,1}(22,:)'"/1 -> dotprod22/1
  dotprod22/1 -> Mux/22
  "IW{2,1}(23,:)'"/1 -> dotprod23/1
  dotprod23/1 -> Mux/23
  "IW{2,1}(24,:)'"/1 -> dotprod24/1
  dotprod24/1 -> Mux/24
  "IW{2,1}(25,:)'"/1 -> dotprod25/1
  dotprod25/1 -> Mux/25
  "IW{2,1}(26,:)'"/1 -> dotprod26/1
  dotprod26/1 -> Mux/26
  "IW{2,1}(27,:)'"/1 -> dotprod27/1
  dotprod27/1 -> Mux/27
  "IW{2,1}(28,:)'"/1 -> dotprod28/1
  dotprod28/1 -> Mux/28
  "IW{2,1}(29,:)'"/1 -> dotprod29/1
  dotprod29/1 -> Mux/29
  "IW{2,1}(30,:)'"/1 -> dotprod30/1
  dotprod30/1 -> Mux/30
  "IW{2,1}(31,:)'"/1 -> dotprod31/1
  dotprod31/1 -> Mux/31
  "IW{2,1}(32,:)'"/1 -> dotprod32/1
  dotprod32/1 -> Mux/32
  "IW{2,1}(33,:)'"/1 -> dotprod33/1
  dotprod33/1 -> Mux/33
  "IW{2,1}(34,:)'"/1 -> dotprod34/1
  dotprod34/1 -> Mux/34
  "IW{2,1}(35,:)'"/1 -> dotprod35/1
  dotprod35/1 -> Mux/35
  "IW{2,1}(36,:)'"/1 -> dotprod36/1
  dotprod36/1 -> Mux/36
  "IW{2,1}(37,:)'"/1 -> dotprod37/1
  dotprod37/1 -> Mux/37
  "IW{2,1}(38,:)'"/1 -> dotprod38/1
  dotprod38/1 -> Mux/38
  "IW{2,1}(39,:)'"/1 -> dotprod39/1
  dotprod39/1 -> Mux/39
  "IW{2,1}(40,:)'"/1 -> dotprod40/1
  dotprod40/1 -> Mux/40
  "IW{2,1}(41,:)'"/1 -> dotprod41/1
  dotprod41/1 -> Mux/41
  "IW{2,1}(42,:)'"/1 -> dotprod42/1
  dotprod42/1 -> Mux/42
  "IW{2,1}(43,:)'"/1 -> dotprod43/1
  dotprod43/1 -> Mux/43
  "IW{2,1}(44,:)'"/1 -> dotprod44/1
  dotprod44/1 -> Mux/44
  "IW{2,1}(45,:)'"/1 -> dotprod45/1
  dotprod45/1 -> Mux/45
  "IW{2,1}(46,:)'"/1 -> dotprod46/1
  dotprod46/1 -> Mux/46
  "IW{2,1}(47,:)'"/1 -> dotprod47/1
  dotprod47/1 -> Mux/47
  "IW{2,1}(48,:)'"/1 -> dotprod48/1
  dotprod48/1 -> Mux/48
  "IW{2,1}(49,:)'"/1 -> dotprod49/1
  dotprod49/1 -> Mux/49
  "IW{2,1}(50,:)'"/1 -> dotprod50/1
  dotprod50/1 -> Mux/50
  "IW{2,1}(51,:)'"/1 -> dotprod51/1
  dotprod51/1 -> Mux/51
  "IW{2,1}(52,:)'"/1 -> dotprod52/1
  dotprod52/1 -> Mux/52
  "IW{2,1}(53,:)'"/1 -> dotprod53/1
  dotprod53/1 -> Mux/53
  "IW{2,1}(54,:)'"/1 -> dotprod54/1
  dotprod54/1 -> Mux/54
  "IW{2,1}(55,:)'"/1 -> dotprod55/1
  dotprod55/1 -> Mux/55
  "IW{2,1}(56,:)'"/1 -> dotprod56/1
  dotprod56/1 -> Mux/56
  "IW{2,1}(57,:)'"/1 -> dotprod57/1
  dotprod57/1 -> Mux/57
  "IW{2,1}(58,:)'"/1 -> dotprod58/1
  dotprod58/1 -> Mux/58
  "IW{2,1}(59,:)'"/1 -> dotprod59/1
  dotprod59/1 -> Mux/59
  "IW{2,1}(60,:)'"/1 -> dotprod60/1
  dotprod60/1 -> Mux/60
  "IW{2,1}(61,:)'"/1 -> dotprod61/1
  dotprod61/1 -> Mux/61
  "IW{2,1}(62,:)'"/1 -> dotprod62/1
  dotprod62/1 -> Mux/62
  "IW{2,1}(63,:)'"/1 -> dotprod63/1
  dotprod63/1 -> Mux/63
  "IW{2,1}(64,:)'"/1 -> dotprod64/1
  dotprod64/1 -> Mux/64
  "IW{2,1}(65,:)'"/1 -> dotprod65/1
  dotprod65/1 -> Mux/65
  "IW{2,1}(66,:)'"/1 -> dotprod66/1
  dotprod66/1 -> Mux/66
  "IW{2,1}(67,:)'"/1 -> dotprod67/1
  dotprod67/1 -> Mux/67
  "IW{2,1}(68,:)'"/1 -> dotprod68/1
  dotprod68/1 -> Mux/68
  "IW{2,1}(69,:)'"/1 -> dotprod69/1
  dotprod69/1 -> Mux/69
  "IW{2,1}(70,:)'"/1 -> dotprod70/1
  dotprod70/1 -> Mux/70
  "IW{2,1}(71,:)'"/1 -> dotprod71/1
  dotprod71/1 -> Mux/71
  "IW{2,1}(72,:)'"/1 -> dotprod72/1
  dotprod72/1 -> Mux/72
  "IW{2,1}(73,:)'"/1 -> dotprod73/1
  dotprod73/1 -> Mux/73
  "IW{2,1}(74,:)'"/1 -> dotprod74/1
  dotprod74/1 -> Mux/74
  "IW{2,1}(75,:)'"/1 -> dotprod75/1
  dotprod75/1 -> Mux/75
  "IW{2,1}(76,:)'"/1 -> dotprod76/1
  dotprod76/1 -> Mux/76
  "IW{2,1}(77,:)'"/1 -> dotprod77/1
  dotprod77/1 -> Mux/77
  "IW{2,1}(78,:)'"/1 -> dotprod78/1
  dotprod78/1 -> Mux/78
  "IW{2,1}(79,:)'"/1 -> dotprod79/1
  dotprod79/1 -> Mux/79
  "IW{2,1}(80,:)'"/1 -> dotprod80/1
  dotprod80/1 -> Mux/80
  "IW{2,1}(81,:)'"/1 -> dotprod81/1
  dotprod81/1 -> Mux/81
  "IW{2,1}(82,:)'"/1 -> dotprod82/1
  dotprod82/1 -> Mux/82
  "IW{2,1}(83,:)'"/1 -> dotprod83/1
  dotprod83/1 -> Mux/83
  "IW{2,1}(84,:)'"/1 -> dotprod84/1
  dotprod84/1 -> Mux/84
  "IW{2,1}(85,:)'"/1 -> dotprod85/1
  dotprod85/1 -> Mux/85
  "IW{2,1}(86,:)'"/1 -> dotprod86/1
  dotprod86/1 -> Mux/86
  "IW{2,1}(87,:)'"/1 -> dotprod87/1
  dotprod87/1 -> Mux/87
  "IW{2,1}(88,:)'"/1 -> dotprod88/1
  dotprod88/1 -> Mux/88
  "IW{2,1}(89,:)'"/1 -> dotprod89/1
  dotprod89/1 -> Mux/89
  "IW{2,1}(90,:)'"/1 -> dotprod90/1
  dotprod90/1 -> Mux/90
  "IW{2,1}(91,:)'"/1 -> dotprod91/1
  dotprod91/1 -> Mux/91
  "IW{2,1}(92,:)'"/1 -> dotprod92/1
  dotprod92/1 -> Mux/92
  "IW{2,1}(93,:)'"/1 -> dotprod93/1
  dotprod93/1 -> Mux/93
  "IW{2,1}(94,:)'"/1 -> dotprod94/1
  dotprod94/1 -> Mux/94
  "IW{2,1}(95,:)'"/1 -> dotprod95/1
  dotprod95/1 -> Mux/95
  "IW{2,1}(96,:)'"/1 -> dotprod96/1
  dotprod96/1 -> Mux/96
  "IW{2,1}(97,:)'"/1 -> dotprod97/1
  dotprod97/1 -> Mux/97
  "IW{2,1}(98,:)'"/1 -> dotprod98/1
  dotprod98/1 -> Mux/98
  "IW{2,1}(99,:)'"/1 -> dotprod99/1
  dotprod99/1 -> Mux/99
  "IW{2,1}(100,:)'"/1 -> dotprod100/1
  dotprod100/1 -> Mux/100
  "IW{2,1}(101,:)'"/1 -> dotprod101/1
  dotprod101/1 -> Mux/101
  "IW{2,1}(102,:)'"/1 -> dotprod102/1
  dotprod102/1 -> Mux/102
  "IW{2,1}(103,:)'"/1 -> dotprod103/1
  dotprod103/1 -> Mux/103
  "IW{2,1}(104,:)'"/1 -> dotprod104/1
  dotprod104/1 -> Mux/104
  "IW{2,1}(105,:)'"/1 -> dotprod105/1
  dotprod105/1 -> Mux/105
  "IW{2,1}(106,:)'"/1 -> dotprod106/1
  dotprod106/1 -> Mux/106
  "IW{2,1}(107,:)'"/1 -> dotprod107/1
  dotprod107/1 -> Mux/107
  "IW{2,1}(108,:)'"/1 -> dotprod108/1
  dotprod108/1 -> Mux/108
  "IW{2,1}(109,:)'"/1 -> dotprod109/1
  dotprod109/1 -> Mux/109
  "IW{2,1}(110,:)'"/1 -> dotprod110/1
  dotprod110/1 -> Mux/110
  "IW{2,1}(111,:)'"/1 -> dotprod111/1
  dotprod111/1 -> Mux/111
  "IW{2,1}(112,:)'"/1 -> dotprod112/1
  dotprod112/1 -> Mux/112
  "IW{2,1}(113,:)'"/1 -> dotprod113/1
  dotprod113/1 -> Mux/113
  "IW{2,1}(114,:)'"/1 -> dotprod114/1
  dotprod114/1 -> Mux/114
  "IW{2,1}(115,:)'"/1 -> dotprod115/1
  dotprod115/1 -> Mux/115
  "IW{2,1}(116,:)'"/1 -> dotprod116/1
  dotprod116/1 -> Mux/116
  "IW{2,1}(117,:)'"/1 -> dotprod117/1
  dotprod117/1 -> Mux/117
  "IW{2,1}(118,:)'"/1 -> dotprod118/1
  dotprod118/1 -> Mux/118
  "IW{2,1}(119,:)'"/1 -> dotprod119/1
  dotprod119/1 -> Mux/119
  "IW{2,1}(120,:)'"/1 -> dotprod120/1
  dotprod120/1 -> Mux/120
  "IW{2,1}(121,:)'"/1 -> dotprod121/1
  dotprod121/1 -> Mux/121
  "IW{2,1}(122,:)'"/1 -> dotprod122/1
  dotprod122/1 -> Mux/122
  "IW{2,1}(123,:)'"/1 -> dotprod123/1
  dotprod123/1 -> Mux/123
  "IW{2,1}(124,:)'"/1 -> dotprod124/1
  dotprod124/1 -> Mux/124
  "IW{2,1}(125,:)'"/1 -> dotprod125/1
  dotprod125/1 -> Mux/125
  "IW{2,1}(126,:)'"/1 -> dotprod126/1
  dotprod126/1 -> Mux/126
  "IW{2,1}(127,:)'"/1 -> dotprod127/1
  dotprod127/1 -> Mux/127
  "IW{2,1}(128,:)'"/1 -> dotprod128/1
  dotprod128/1 -> Mux/128
  "IW{2,1}(129,:)'"/1 -> dotprod129/1
  dotprod129/1 -> Mux/129
  "IW{2,1}(130,:)'"/1 -> dotprod130/1
  dotprod130/1 -> Mux/130
  "IW{2,1}(131,:)'"/1 -> dotprod131/1
  dotprod131/1 -> Mux/131
  "IW{2,1}(132,:)'"/1 -> dotprod132/1
  dotprod132/1 -> Mux/132
  "IW{2,1}(133,:)'"/1 -> dotprod133/1
  dotprod133/1 -> Mux/133
  "IW{2,1}(134,:)'"/1 -> dotprod134/1
  dotprod134/1 -> Mux/134
  "IW{2,1}(135,:)'"/1 -> dotprod135/1
  dotprod135/1 -> Mux/135
  "IW{2,1}(136,:)'"/1 -> dotprod136/1
  dotprod136/1 -> Mux/136
  "IW{2,1}(137,:)'"/1 -> dotprod137/1
  dotprod137/1 -> Mux/137
  "IW{2,1}(138,:)'"/1 -> dotprod138/1
  dotprod138/1 -> Mux/138
  "IW{2,1}(139,:)'"/1 -> dotprod139/1
  dotprod139/1 -> Mux/139
  "IW{2,1}(140,:)'"/1 -> dotprod140/1
  dotprod140/1 -> Mux/140
  "IW{2,1}(141,:)'"/1 -> dotprod141/1
  dotprod141/1 -> Mux/141
  "IW{2,1}(142,:)'"/1 -> dotprod142/1
  dotprod142/1 -> Mux/142
  "IW{2,1}(143,:)'"/1 -> dotprod143/1
  dotprod143/1 -> Mux/143
  "IW{2,1}(144,:)'"/1 -> dotprod144/1
  dotprod144/1 -> Mux/144
  "IW{2,1}(145,:)'"/1 -> dotprod145/1
  dotprod145/1 -> Mux/145
  "IW{2,1}(146,:)'"/1 -> dotprod146/1
  dotprod146/1 -> Mux/146
  "IW{2,1}(147,:)'"/1 -> dotprod147/1
  dotprod147/1 -> Mux/147
  "IW{2,1}(148,:)'"/1 -> dotprod148/1
  dotprod148/1 -> Mux/148
  "IW{2,1}(149,:)'"/1 -> dotprod149/1
  dotprod149/1 -> Mux/149
  "IW{2,1}(150,:)'"/1 -> dotprod150/1
  dotprod150/1 -> Mux/150
  "IW{2,1}(151,:)'"/1 -> dotprod151/1
  dotprod151/1 -> Mux/151
  "IW{2,1}(152,:)'"/1 -> dotprod152/1
  dotprod152/1 -> Mux/152
  "IW{2,1}(153,:)'"/1 -> dotprod153/1
  dotprod153/1 -> Mux/153
  "IW{2,1}(154,:)'"/1 -> dotprod154/1
  dotprod154/1 -> Mux/154
  "IW{2,1}(155,:)'"/1 -> dotprod155/1
  dotprod155/1 -> Mux/155
  "IW{2,1}(156,:)'"/1 -> dotprod156/1
  dotprod156/1 -> Mux/156
  "IW{2,1}(157,:)'"/1 -> dotprod157/1
  dotprod157/1 -> Mux/157
  "IW{2,1}(158,:)'"/1 -> dotprod158/1
  dotprod158/1 -> Mux/158
  "IW{2,1}(159,:)'"/1 -> dotprod159/1
  dotprod159/1 -> Mux/159
  "IW{2,1}(160,:)'"/1 -> dotprod160/1
  dotprod160/1 -> Mux/160
  "IW{2,1}(161,:)'"/1 -> dotprod161/1
  dotprod161/1 -> Mux/161
  "IW{2,1}(162,:)'"/1 -> dotprod162/1
  dotprod162/1 -> Mux/162
  "IW{2,1}(163,:)'"/1 -> dotprod163/1
  dotprod163/1 -> Mux/163
  "IW{2,1}(164,:)'"/1 -> dotprod164/1
  dotprod164/1 -> Mux/164
  "IW{2,1}(165,:)'"/1 -> dotprod165/1
  dotprod165/1 -> Mux/165
  "IW{2,1}(166,:)'"/1 -> dotprod166/1
  dotprod166/1 -> Mux/166
  "IW{2,1}(167,:)'"/1 -> dotprod167/1
  dotprod167/1 -> Mux/167
  "IW{2,1}(168,:)'"/1 -> dotprod168/1
  dotprod168/1 -> Mux/168
  "IW{2,1}(169,:)'"/1 -> dotprod169/1
  dotprod169/1 -> Mux/169
  "IW{2,1}(170,:)'"/1 -> dotprod170/1
  dotprod170/1 -> Mux/170
  "IW{2,1}(171,:)'"/1 -> dotprod171/1
  dotprod171/1 -> Mux/171
  "IW{2,1}(172,:)'"/1 -> dotprod172/1
  dotprod172/1 -> Mux/172
  "IW{2,1}(173,:)'"/1 -> dotprod173/1
  dotprod173/1 -> Mux/173
  "IW{2,1}(174,:)'"/1 -> dotprod174/1
  dotprod174/1 -> Mux/174
  "IW{2,1}(175,:)'"/1 -> dotprod175/1
  dotprod175/1 -> Mux/175
  "IW{2,1}(176,:)'"/1 -> dotprod176/1
  dotprod176/1 -> Mux/176
  "IW{2,1}(177,:)'"/1 -> dotprod177/1
  dotprod177/1 -> Mux/177
  "IW{2,1}(178,:)'"/1 -> dotprod178/1
  dotprod178/1 -> Mux/178
  "IW{2,1}(179,:)'"/1 -> dotprod179/1
  dotprod179/1 -> Mux/179
  "IW{2,1}(180,:)'"/1 -> dotprod180/1
  dotprod180/1 -> Mux/180
  "IW{2,1}(181,:)'"/1 -> dotprod181/1
  dotprod181/1 -> Mux/181
  "IW{2,1}(182,:)'"/1 -> dotprod182/1
  dotprod182/1 -> Mux/182
  "IW{2,1}(183,:)'"/1 -> dotprod183/1
  dotprod183/1 -> Mux/183
  "IW{2,1}(184,:)'"/1 -> dotprod184/1
  dotprod184/1 -> Mux/184
  "IW{2,1}(185,:)'"/1 -> dotprod185/1
  dotprod185/1 -> Mux/185
  "IW{2,1}(186,:)'"/1 -> dotprod186/1
  dotprod186/1 -> Mux/186
  "IW{2,1}(187,:)'"/1 -> dotprod187/1
  dotprod187/1 -> Mux/187
  "IW{2,1}(188,:)'"/1 -> dotprod188/1
  dotprod188/1 -> Mux/188
  "IW{2,1}(189,:)'"/1 -> dotprod189/1
  dotprod189/1 -> Mux/189
  "IW{2,1}(190,:)'"/1 -> dotprod190/1
  dotprod190/1 -> Mux/190
  "IW{2,1}(191,:)'"/1 -> dotprod191/1
  dotprod191/1 -> Mux/191
  "IW{2,1}(192,:)'"/1 -> dotprod192/1
  dotprod192/1 -> Mux/192
  "IW{2,1}(193,:)'"/1 -> dotprod193/1
  dotprod193/1 -> Mux/193
  "IW{2,1}(194,:)'"/1 -> dotprod194/1
  dotprod194/1 -> Mux/194
  "IW{2,1}(195,:)'"/1 -> dotprod195/1
  dotprod195/1 -> Mux/195
  "IW{2,1}(196,:)'"/1 -> dotprod196/1
  dotprod196/1 -> Mux/196
  "IW{2,1}(197,:)'"/1 -> dotprod197/1
  dotprod197/1 -> Mux/197
  "IW{2,1}(198,:)'"/1 -> dotprod198/1
  dotprod198/1 -> Mux/198
  "IW{2,1}(199,:)'"/1 -> dotprod199/1
  dotprod199/1 -> Mux/199
  "IW{2,1}(200,:)'"/1 -> dotprod200/1
  dotprod200/1 -> Mux/200
  Mux/1 -> "lz{2,1}"/1
